simulink model "power_switch"  (R2020a)
settings: Solver=VariableStepAuto  StartTime=0.0  StopTime=1000  RelTol=1e-3
libraries: xpcutilitieslib x3, xpcrtudplib x2, lib_header_20a x1, lib_subframe_20a x1
settings Model: EnablePacing=on  PacingRate=0.010000  Creator=han22004  LastModifiedBy=han22004

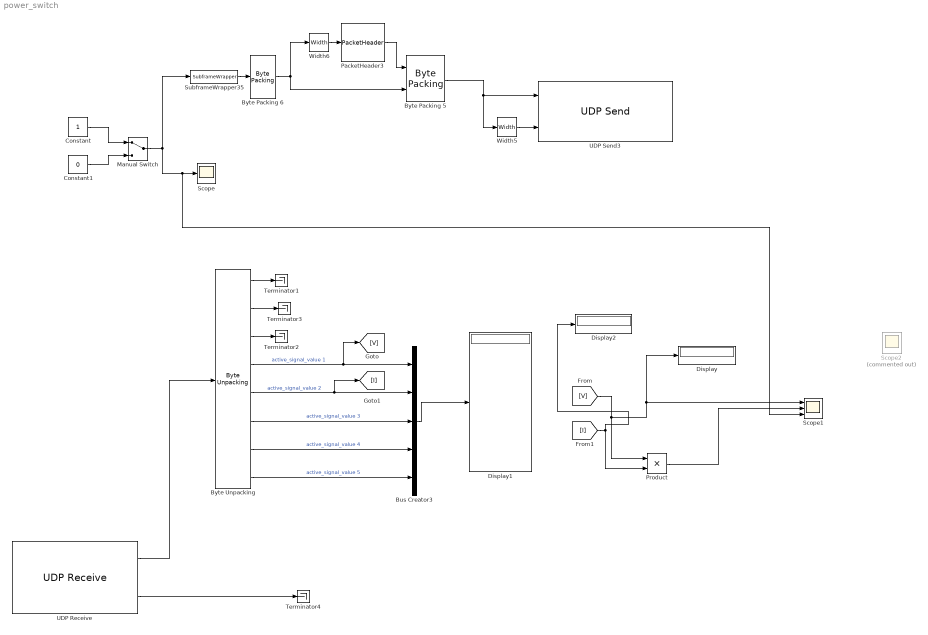
== system power_switch ==
  Bus Creator3 : BusCreator  Inputs=5
  Byte Packing 5 : xpcutilitieslib/Byte Packing   MaskPackedDataType=uint8  MaskUnpackedDataTypes={'uint8', 'uint8'}  MaskAlignment=1
  Byte Packing 6 : xpcutilitieslib/Byte Packing   MaskPackedDataType=uint8  MaskUnpackedDataTypes={'uint8'}  MaskAlignment=1
  "Byte Unpacking " : xpcutilitieslib/Byte Unpacking   MaskUnpackedDataTypes={'uint8','uint16','uint8','double','double','double','double','double'}  MaskUnpackedDataSizes={[22],[1],[6],[1],[1],[1],[1],[1]}  MaskAlignment=1
      settings: SourceProductBaseCode=XP
  Constant : Constant  SampleTime=0.01
  Constant1 : Constant  Value=0  SampleTime=0.01
  Display : Display
  Display1 : Display
      settings: Format=decimal (Stored Integer)
  Display2 : Display
  Manual Switch : ManualSwitch
  PacketHeader3 : lib_header_20a/PacketHeader  src=8  dst=1  pkt_type=1  pkt_priority=0  service=0  flag=0  option1=0  option2=0  subframe_num=1
  Product : Product
  Scope : Scope
  Scope1 : Scope  NumInputPorts=3
  Scope2 : Scope  Commented=on  NumInputPorts=3
  SubframeWrapper35 : lib_subframe_20a/SubframeWrapper  data_id=1234
  Terminator{1..4} (4 alike) : Terminator
  UDP Receive : xpcrtudplib/UDP Receive  ipAddressVal=Use host-target connection  localPort=12345  rcvWidth=30 + 8 * 5  rcvFmAny=on  fmAddress=0.0.0.0  rcvMulticast=off  multicastAddress={}  maxUDPQueue=8  sampleTime=-1
  UDP Send3 : xpcrtudplib/UDP Send  ipAddressVal=Use host-target connection  localPort=-1  toAddress=192.168.0.12  toPort=12345  sampleTime=-1
      settings: SourceProductBaseCode=XP
  Width5 : Width
  Width6 : Width
  wires:
  Width5/1 -> UDP Send3/2
  PacketHeader3/1 -> Byte Packing 5/1
  Byte Packing 6/1 -> Width6/1, Byte Packing 5/2
  Byte Packing 5/1 -> Width5/1, UDP Send3/1
  Width6/1 -> PacketHeader3/1
  SubframeWrapper35/1 -> Byte Packing 6/1
  Manual Switch/1 -> Scope1/3, Scope/1, SubframeWrapper35/1
  Constant/1 -> Manual Switch/1
  Constant1/1 -> Manual Switch/2
  "Byte Unpacking "/5 -> [I], Bus Creator3/2  "active_signal_value 2"
  "Byte Unpacking "/1 -> Terminator1/1
  "Byte Unpacking "/7 -> Bus Creator3/4  "active_signal_value 4"
  "Byte Unpacking "/6 -> Bus Creator3/3  "active_signal_value 3"
  "Byte Unpacking "/8 -> Bus Creator3/5  "active_signal_value 5"
  UDP Receive/1 -> "Byte Unpacking "/1
  "Byte Unpacking "/3 -> Terminator2/1
  "Byte Unpacking "/4 -> [V], Bus Creator3/1  "active_signal_value 1"
  "Byte Unpacking "/2 -> Terminator3/1
  UDP Receive/2 -> Terminator4/1
  Bus Creator3/1 -> Display1/1
  [V] -> Product/1, Scope1/1, Display/1
  [I] -> Product/2, Display2/1
  Product/1 -> Scope1/2
